simulink model "SystummThinkers_Simulink"  (R2025a)
settings: Solver=VariableStepAuto  StartTime=0.0  StopTime=50  RelTol=1e-3
libraries: slpidlib x2
settings Model: Creator=mostlyk  LastModifiedBy=Anish Toshniwal

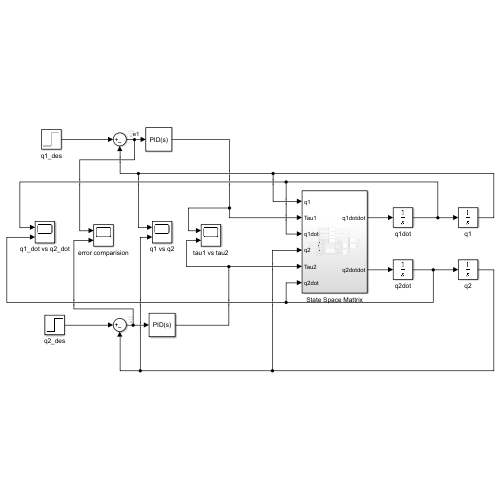
[thumbnail: Simulink's stored preview of the top-level diagram]
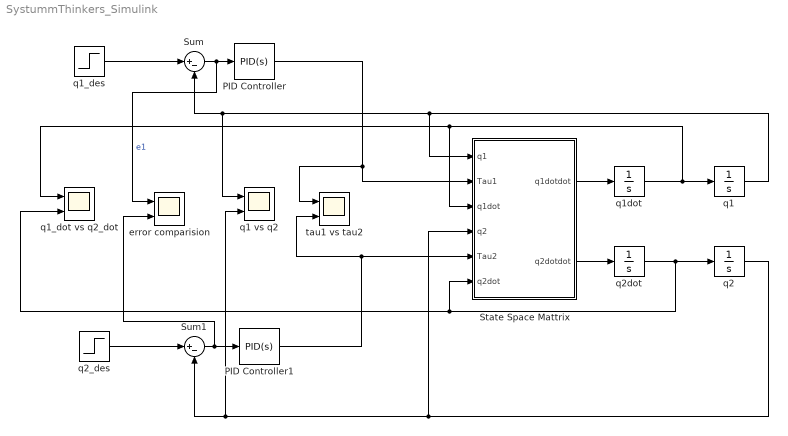
== system SystummThinkers_Simulink ==
  PID Controller : slpidlib/PID Controller  Controller=PID  Form=Parallel  TimeDomain=Continuous-time  UseExternalTs=off  SampleTime=-1  IntegratorMethod=Forward Euler  FilterMethod=Forward Euler  ControllerParametersSource=internal  P=120  I=180  UseKiTs=off  D=150  UseExternalDerivativeSource=off  N=100  UseFilter=on  TunerSelectOption=Transfer Function Based (PID Tuner App)  InitialConditionSource=internal  InitialConditionForIntegrator=0  InitialConditionForFilter=0  DifferentiatorICPrevScaledInput=0  ExternalReset=none  TrackingMode=off  Kt=1  LimitOutput=off  SatLimitsSource=internal  UpperSaturationLimit=inf  LowerSaturationLimit=-inf  LinearizeAsGain=on  AntiWindupMode=none  Kb=1  LimitIntegrator=off  UpperIntegratorSaturationLimit=inf  LowerIntegratorSaturationLimit=-inf  POutMin=[]  POutMax=[]  IOutMin=[]  IOutMax=[]  DOutMin=[]  DOutMax=[]  NOutMin=[]  NOutMax=[]  SumOutMin=[]  SumOutMax=[]  SaturationOutMin=[]  SaturationOutMax=[]  PParamMin=[]  PParamMax=[]  IParamMin=[]  IParamMax=[]  DParamMin=[]  DParamMax=[]  NParamMin=[]  NParamMax=[]  KbParamMin=[]  KbParamMax=[]  KtParamMin=[]  KtParamMax=[]  KbOutMin=[]  KbOutMax=[]  KtOutMin=[]  KtOutMax=[]  IntegratorOutMin=[]  IntegratorOutMax=[]  FilterOutMin=[]  FilterOutMax=[]  SumI1OutMin=[]  SumI1OutMax=[]  SumI2OutMin=[]  SumI2OutMax=[]  SumI3OutMin=[]  SumI3OutMax=[]  SumI4OutMin=[]  SumI4OutMax=[]  SumDOutMin=[]  SumDOutMax=[]  DifferentiatorOutMin=[]  DifferentiatorOutMax=[]  FilterDiffOutCoefMin=[]  FilterDiffOutCoefMax=[]  ReciprocalOutMin=[]  ReciprocalOutMax=[]  SumDenOutMin=[]  SumDenOutMax=[]  SumNumOutMin=[]  SumNumOutMax=[]  DivideOutMin=[]  DivideOutMax=[]  UdiffTsProdOutMin=[]  UdiffTsProdOutMax=[]  NTsProdOutMin=[]  NTsProdOutMax=[]  UintegralTsProdOutMin=[]  UintegralTsProdOutMax=[]  UngainTsProdOutMin=[]  UngainTsProdOutMax=[]  ClampingZeroOutDataTypeStr=Inherit: Inherit via back propagation  ClampingZeroOutMin=[]  ClampingZeroOutMax=[]  FilterDenConstantOutDataTypeStr=Inherit: Inherit via back propagation  FilterDenConstantOutMin=[]  FilterDenConstantOutMax=[]  PCopyOutDataTypeStr=Inherit: Inherit via back propagation  PCopyOutMin=[]  PCopyOutMax=[]  NCopyOutDataTypeStr=Inherit: Inherit via back propagation  NCopyOutMin=[]  NCopyOutMax=[]  IntegratorContinuousStateAttributes=''  IntegratorStateMustResolveToSignalObject=off  IntegratorRTWStateStorageClass=Auto  FilterContinuousStateAttributes=''  FilterStateMustResolveToSignalObject=off  FilterRTWStateStorageClass=Auto  ParallelPVariant=InternalParameters  IdealPVariant=Disabled  IVariant=InternalParameters  DVariant=InternalParameters  IntegratorVariant=Continuous  SatVariant=Disabled  AWVariant=Passthrough  PCopyVariant=Disabled  TRVariant=Disabled  FdbkBlocksVariant=Forward  IdealPFdbkVariant=Disabled  SatFdbkVariant=Disabled  DerivativeFilterVariant=ContFilter  NVariant=InternalParameters  NCopyVariant=Disabled  FilterICVariant=InternalICsFilter  IntegratorICVariant=InternalICs  ExternalResetVariant=Disabled  TRSumVariant=Passthrough  SumFdbkVariant=Disabled  SumVariant=Sum_PID  TsampFilterVariant=InternalTs  TsampNgainVariant=Passthrough  TsampIntegralVariant=Disabled_SignalSpec  ExternalSaturationOutDataTypeStr=Inherit: Same as second input  DerivativeSourceVariant=ErrorSignal  PreIntVariant=InternalPreInt
  PID Controller1 : slpidlib/PID Controller  Controller=PID  Form=Parallel  TimeDomain=Continuous-time  UseExternalTs=off  SampleTime=-1  IntegratorMethod=Forward Euler  FilterMethod=Forward Euler  ControllerParametersSource=internal  P=120  I=180  UseKiTs=off  D=150  UseExternalDerivativeSource=off  N=100  UseFilter=on  TunerSelectOption=Transfer Function Based (PID Tuner App)  InitialConditionSource=internal  InitialConditionForIntegrator=0  InitialConditionForFilter=0  DifferentiatorICPrevScaledInput=0  ExternalReset=none  TrackingMode=off  Kt=1  LimitOutput=off  SatLimitsSource=internal  UpperSaturationLimit=inf  LowerSaturationLimit=-inf  LinearizeAsGain=on  AntiWindupMode=none  Kb=1  LimitIntegrator=off  UpperIntegratorSaturationLimit=inf  LowerIntegratorSaturationLimit=-inf  POutMin=[]  POutMax=[]  IOutMin=[]  IOutMax=[]  DOutMin=[]  DOutMax=[]  NOutMin=[]  NOutMax=[]  SumOutMin=[]  SumOutMax=[]  SaturationOutMin=[]  SaturationOutMax=[]  PParamMin=[]  PParamMax=[]  IParamMin=[]  IParamMax=[]  DParamMin=[]  DParamMax=[]  NParamMin=[]  NParamMax=[]  KbParamMin=[]  KbParamMax=[]  KtParamMin=[]  KtParamMax=[]  KbOutMin=[]  KbOutMax=[]  KtOutMin=[]  KtOutMax=[]  IntegratorOutMin=[]  IntegratorOutMax=[]  FilterOutMin=[]  FilterOutMax=[]  SumI1OutMin=[]  SumI1OutMax=[]  SumI2OutMin=[]  SumI2OutMax=[]  SumI3OutMin=[]  SumI3OutMax=[]  SumI4OutMin=[]  SumI4OutMax=[]  SumDOutMin=[]  SumDOutMax=[]  DifferentiatorOutMin=[]  DifferentiatorOutMax=[]  FilterDiffOutCoefMin=[]  FilterDiffOutCoefMax=[]  ReciprocalOutMin=[]  ReciprocalOutMax=[]  SumDenOutMin=[]  SumDenOutMax=[]  SumNumOutMin=[]  SumNumOutMax=[]  DivideOutMin=[]  DivideOutMax=[]  UdiffTsProdOutMin=[]  UdiffTsProdOutMax=[]  NTsProdOutMin=[]  NTsProdOutMax=[]  UintegralTsProdOutMin=[]  UintegralTsProdOutMax=[]  UngainTsProdOutMin=[]  UngainTsProdOutMax=[]  ClampingZeroOutDataTypeStr=Inherit: Inherit via back propagation  ClampingZeroOutMin=[]  ClampingZeroOutMax=[]  FilterDenConstantOutDataTypeStr=Inherit: Inherit via back propagation  FilterDenConstantOutMin=[]  FilterDenConstantOutMax=[]  PCopyOutDataTypeStr=Inherit: Inherit via back propagation  PCopyOutMin=[]  PCopyOutMax=[]  NCopyOutDataTypeStr=Inherit: Inherit via back propagation  NCopyOutMin=[]  NCopyOutMax=[]  IntegratorContinuousStateAttributes=''  IntegratorStateMustResolveToSignalObject=off  IntegratorRTWStateStorageClass=Auto  FilterContinuousStateAttributes=''  FilterStateMustResolveToSignalObject=off  FilterRTWStateStorageClass=Auto  ParallelPVariant=InternalParameters  IdealPVariant=Disabled  IVariant=InternalParameters  DVariant=InternalParameters  IntegratorVariant=Continuous  SatVariant=Disabled  AWVariant=Passthrough  PCopyVariant=Disabled  TRVariant=Disabled  FdbkBlocksVariant=Forward  IdealPFdbkVariant=Disabled  SatFdbkVariant=Disabled  DerivativeFilterVariant=ContFilter  NVariant=InternalParameters  NCopyVariant=Disabled  FilterICVariant=InternalICsFilter  IntegratorICVariant=InternalICs  ExternalResetVariant=Disabled  TRSumVariant=Passthrough  SumFdbkVariant=Disabled  SumVariant=Sum_PID  TsampFilterVariant=InternalTs  TsampNgainVariant=Passthrough  TsampIntegralVariant=Disabled_SignalSpec  ExternalSaturationOutDataTypeStr=Inherit: Same as second input  DerivativeSourceVariant=ErrorSignal  PreIntVariant=InternalPreInt
  State Space Mattrix : Subsystem
  Sum : Sum  Inputs=|+-
  Sum1 : Sum  Inputs=|+-
  error comparision : Scope  NumInputPorts=2
      settings: ActiveDisplayYMinimum=-1  ActiveDisplayYMaximum=1
  q1 : Integrator  InitialCondition=0.1
  q1 vs q2 : Scope  NumInputPorts=2
      settings: ActiveDisplayYMinimum=-0.27365843091544217  ActiveDisplayYMaximum=0.20860466599804511
  q1_des : Step  After=0  SampleTime=0
  q1_dot vs q2_dot : Scope  NumInputPorts=2
      settings: ActiveDisplayYMinimum=-16.221672111581775  ActiveDisplayYMaximum=9.3160134029449342  DataLoggingVariableName=ScopeData2
  q1dot : Integrator
  q2 : Integrator  InitialCondition=0.1
  q2_des : Step  After=0  SampleTime=0
  q2dot : Integrator
  tau1 vs tau2 : Scope  NumInputPorts=2
      settings: ActiveDisplayYMinimum=-30.7924543124781  ActiveDisplayYMaximum=40.414840154467996  DataLoggingVariableName=ScopeData3
  wires:
  q1/1 -> State Space Mattrix/1(q1), Sum/2, q1 vs q2/1
  Sum/1 -> PID Controller/1, error comparision/1  "e1"
  q1_des/1 -> Sum/1
  q1dot/1 -> q1_dot vs q2_dot/1, State Space Mattrix/3(q1dot), q1/1
  PID Controller/1 -> tau1 vs tau2/1, State Space Mattrix/2(Tau1)
  q2_des/1 -> Sum1/1
  q2/1 -> Sum1/2, q1 vs q2/2, State Space Mattrix/4(q2)
  State Space Mattrix/2(q2dotdot) -> q2dot/1
  q2dot/1 -> q2/1, q1_dot vs q2_dot/2, State Space Mattrix/6(q2dot)
  PID Controller1/1 -> tau1 vs tau2/2, State Space Mattrix/5(Tau2)
  State Space Mattrix/1(q1dotdot) -> q1dot/1
  Sum1/1 -> error comparision/2, PID Controller1/1

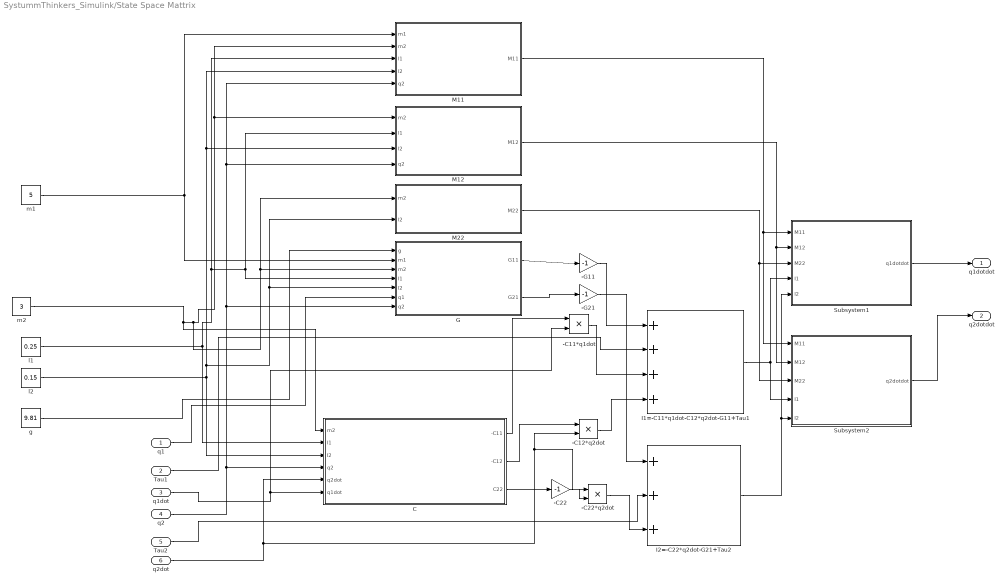
== system SystummThinkers_Simulink/State Space Mattrix ==
  q1 : Inport
  Tau1 : Inport  Port=2
  q1dot : Inport  Port=3
  q2 : Inport  Port=4
  Tau2 : Inport  Port=5
  q2dot : Inport  Port=6
  -C11*q1dot : Product
  -C12*q2dot : Product
  -C22 : Gain  Gain=-1
  -C22*q2dot : Product
  -G11 : Gain  Gain=-1
  -G21 : Gain  Gain=-1
  C : Subsystem
  G : Subsystem
  I1=-C11*q1dot-C12*q2dot-G11+Tau1 : Sum  Inputs=++++
  I2=-C22*q2dot-G21+Tau2 : Sum  Inputs=+++
  M11 : Subsystem
  M12 : Subsystem
  M22 : Subsystem
  Subsystem1 : Subsystem
  Subsystem2 : Subsystem
  g : Constant  Value=9.81
  l1 : Constant  Value=0.25
  l2 : Constant  Value=0.15
  m1 : Constant  Value=5
  m2 : Constant  Value=3
  q1dotdot : Outport
  q2dotdot : Outport  Port=2
  wires:
  m1/1 -> G/2(m1), M11/1(m1)
  m2/1 -> C/1(m2), M22/1(m2), G/3(m2), M11/2(m2), M12/1(m2)
  l1/1 -> C/2(l1), M11/3(l1), G/4(l1), M12/2(l1)
  l2/1 -> C/3(I2), M22/2(l2), G/5(l2), M11/4(l2), M12/3(l2)
  q2/1 -> M11/5(q2), M12/4(q2), G/7(q2), C/4(q2)
  q1/1 -> G/6(q1)
  g/1 -> G/1(g)
  q2dot/1 -> C/5(q2dot), -C12*q2dot/2, -C22*q2dot/1
  q1dot/1 -> -C11*q1dot/2, C/6(q1dot)
  C/1(-C11) -> -C11*q1dot/1
  C/2(-C12) -> -C12*q2dot/1
  G/1(G11) -> -G11/1
  -C12*q2dot/1 -> I1=-C11*q1dot-C12*q2dot-G11+Tau1/4
  -C11*q1dot/1 -> I1=-C11*q1dot-C12*q2dot-G11+Tau1/3
  -G11/1 -> I1=-C11*q1dot-C12*q2dot-G11+Tau1/1
  Tau1/1 -> I1=-C11*q1dot-C12*q2dot-G11+Tau1/2
  C/3(C22) -> -C22/1
  -C22/1 -> -C22*q2dot/2
  G/2(G21) -> -G21/1
  -C22*q2dot/1 -> I2=-C22*q2dot-G21+Tau2/3
  -G21/1 -> I2=-C22*q2dot-G21+Tau2/1
  Tau2/1 -> I2=-C22*q2dot-G21+Tau2/2
  M11/1(M11) -> Subsystem2/1(M11), Subsystem1/1(M11)
  M12/1(M12) -> Subsystem2/2(M12), Subsystem1/2(M12)
  M22/1(M22) -> Subsystem2/3(M22), Subsystem1/3(M22)
  I1=-C11*q1dot-C12*q2dot-G11+Tau1/1 -> Subsystem1/4(I1), Subsystem2/4(I1)
  I2=-C22*q2dot-G21+Tau2/1 -> Subsystem1/5(I2), Subsystem2/5(I2)
  Subsystem1/1("q1dotdot ") -> q1dotdot/1
  Subsystem2/1("q2dotdot ") -> q2dotdot/1

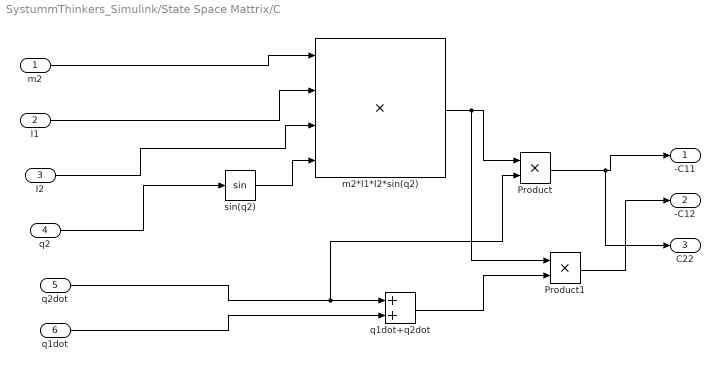
== system SystummThinkers_Simulink/State Space Mattrix/C ==
  m2 : Inport
  l1 : Inport  Port=2
  I2 : Inport  Port=3
  q2 : Inport  Port=4
  q2dot : Inport  Port=5
  q1dot : Inport  Port=6
  Product : Product
  Product1 : Product
  m2*l1*l2*sin(q2) : Product  Inputs=4
  q1dot+q2dot : Sum
  sin(q2) : Trigonometry
  -C11 : Outport
  -C12 : Outport  Port=2
  C22 : Outport  Port=3
  wires:
  q2/1 -> sin(q2)/1
  sin(q2)/1 -> m2*l1*l2*sin(q2)/4
  m2/1 -> m2*l1*l2*sin(q2)/1
  l1/1 -> m2*l1*l2*sin(q2)/2
  I2/1 -> m2*l1*l2*sin(q2)/3
  q1dot/1 -> q1dot+q2dot/2
  q2dot/1 -> Product/2, q1dot+q2dot/1
  m2*l1*l2*sin(q2)/1 -> Product1/1, Product/1
  Product/1 -> C22/1, -C11/1
  q1dot+q2dot/1 -> Product1/2
  Product1/1 -> -C12/1

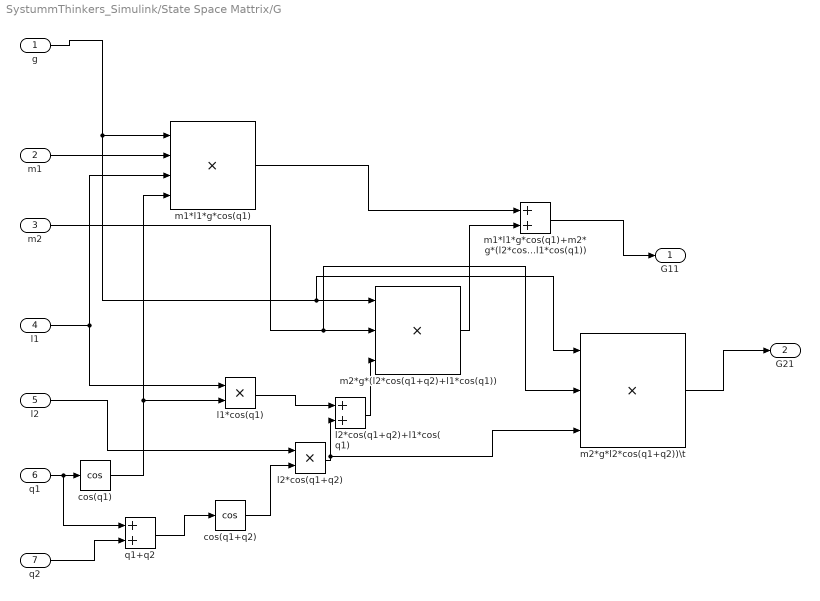
== system SystummThinkers_Simulink/State Space Mattrix/G ==
  g : Inport
  m1 : Inport  Port=2
  m2 : Inport  Port=3
  l1 : Inport  Port=4
  l2 : Inport  Port=5
  q1 : Inport  Port=6
  q2 : Inport  Port=7
  cos(q1) : Trigonometry  Operator=cos
  cos(q1+q2) : Trigonometry  Operator=cos
  l1*cos(q1) : Product
  l2*cos(q1+q2) : Product
  l2*cos(q1+q2)+l1*cos(q1) : Sum
  m1*l1*g*cos(q1) : Product  Inputs=4
  m1*l1*g*cos(q1)+m2*g*(l2*cos(q1+q2)+l1*cos(q1)) : Sum
  m2*g*(l2*cos(q1+q2)+l1*cos(q1)) : Product  Inputs=3
  m2*g*l2*cos(q1+q2))\t : Product  Inputs=3
  q1+q2 : Sum
  G11 : Outport
  G21 : Outport  Port=2
  wires:
  q1/1 -> q1+q2/1, cos(q1)/1
  g/1 -> m2*g*l2*cos(q1+q2))\t/1, m2*g*(l2*cos(q1+q2)+l1*cos(q1))/1, m1*l1*g*cos(q1)/1
  m1/1 -> m1*l1*g*cos(q1)/2
  l1/1 -> l1*cos(q1)/1, m1*l1*g*cos(q1)/3
  cos(q1)/1 -> l1*cos(q1)/2, m1*l1*g*cos(q1)/4
  q2/1 -> q1+q2/2
  q1+q2/1 -> cos(q1+q2)/1
  cos(q1+q2)/1 -> l2*cos(q1+q2)/2
  l2/1 -> l2*cos(q1+q2)/1
  l2*cos(q1+q2)/1 -> m2*g*l2*cos(q1+q2))\t/3, l2*cos(q1+q2)+l1*cos(q1)/2
  l1*cos(q1)/1 -> l2*cos(q1+q2)+l1*cos(q1)/1
  l2*cos(q1+q2)+l1*cos(q1)/1 -> m2*g*(l2*cos(q1+q2)+l1*cos(q1))/3
  m2/1 -> m2*g*(l2*cos(q1+q2)+l1*cos(q1))/2, m2*g*l2*cos(q1+q2))\t/2
  m1*l1*g*cos(q1)/1 -> m1*l1*g*cos(q1)+m2*g*(l2*cos(q1+q2)+l1*cos(q1))/1
  m2*g*(l2*cos(q1+q2)+l1*cos(q1))/1 -> m1*l1*g*cos(q1)+m2*g*(l2*cos(q1+q2)+l1*cos(q1))/2
  m1*l1*g*cos(q1)+m2*g*(l2*cos(q1+q2)+l1*cos(q1))/1 -> G11/1
  m2*g*l2*cos(q1+q2))\t/1 -> G21/1

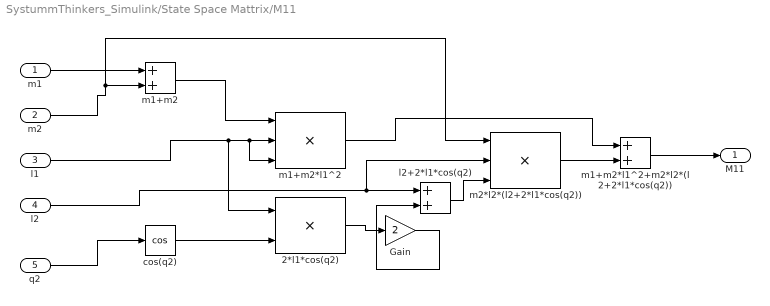
== system SystummThinkers_Simulink/State Space Mattrix/M11 ==
  m1 : Inport
  m2 : Inport  Port=2
  l1 : Inport  Port=3
  l2 : Inport  Port=4
  q2 : Inport  Port=5
  2*l1*cos(q2) : Product
  Gain : Gain  Gain=2
  cos(q2) : Trigonometry  Operator=cos
  l2+2*l1*cos(q2) : Sum
  m1+m2 : Sum
  m1+m2*l1^2 : Product  Inputs=3
  m1+m2*l1^2+m2*l2*(l2+2*l1*cos(q2)) : Sum
  m2*l2*(l2+2*l1*cos(q2)) : Product  Inputs=3
  M11 : Outport
  wires:
  m1/1 -> m1+m2/1
  m2/1 -> m2*l2*(l2+2*l1*cos(q2))/1, m1+m2/2
  m1+m2/1 -> m1+m2*l1^2/1
  l1/1 -> 2*l1*cos(q2)/1, m1+m2*l1^2/3, m1+m2*l1^2/2
  q2/1 -> cos(q2)/1
  cos(q2)/1 -> 2*l1*cos(q2)/2
  l2/1 -> m2*l2*(l2+2*l1*cos(q2))/2, l2+2*l1*cos(q2)/1
  l2+2*l1*cos(q2)/1 -> m2*l2*(l2+2*l1*cos(q2))/3
  m2*l2*(l2+2*l1*cos(q2))/1 -> m1+m2*l1^2+m2*l2*(l2+2*l1*cos(q2))/2
  m1+m2*l1^2/1 -> m1+m2*l1^2+m2*l2*(l2+2*l1*cos(q2))/1
  m1+m2*l1^2+m2*l2*(l2+2*l1*cos(q2))/1 -> M11/1
  2*l1*cos(q2)/1 -> Gain/1
  Gain/1 -> l2+2*l1*cos(q2)/2

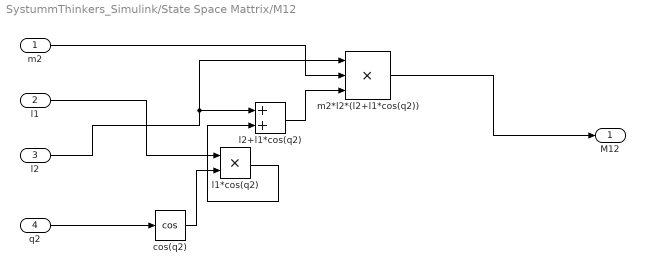
== system SystummThinkers_Simulink/State Space Mattrix/M12 ==
  m2 : Inport
  l1 : Inport  Port=2
  l2 : Inport  Port=3
  q2 : Inport  Port=4
  cos(q2) : Trigonometry  Operator=cos
  l1*cos(q2) : Product
  l2+l1*cos(q2) : Sum
  m2*l2*(l2+l1*cos(q2)) : Product  Inputs=3
  M12 : Outport
  wires:
  q2/1 -> cos(q2)/1
  l1/1 -> l1*cos(q2)/1
  cos(q2)/1 -> l1*cos(q2)/2
  l1*cos(q2)/1 -> l2+l1*cos(q2)/2
  l2/1 -> m2*l2*(l2+l1*cos(q2))/1, l2+l1*cos(q2)/1
  l2+l1*cos(q2)/1 -> m2*l2*(l2+l1*cos(q2))/3
  m2/1 -> m2*l2*(l2+l1*cos(q2))/2
  m2*l2*(l2+l1*cos(q2))/1 -> M12/1

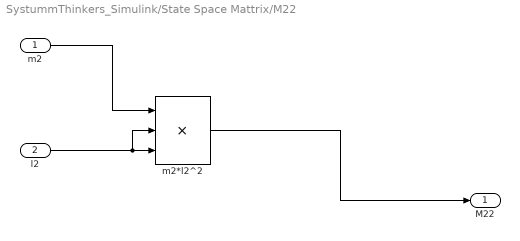
== system SystummThinkers_Simulink/State Space Mattrix/M22 ==
  m2 : Inport
  l2 : Inport  Port=2
  m2*l2^2 : Product  Inputs=3
  M22 : Outport
  wires:
  m2/1 -> m2*l2^2/1
  l2/1 -> m2*l2^2/2, m2*l2^2/3
  m2*l2^2/1 -> M22/1

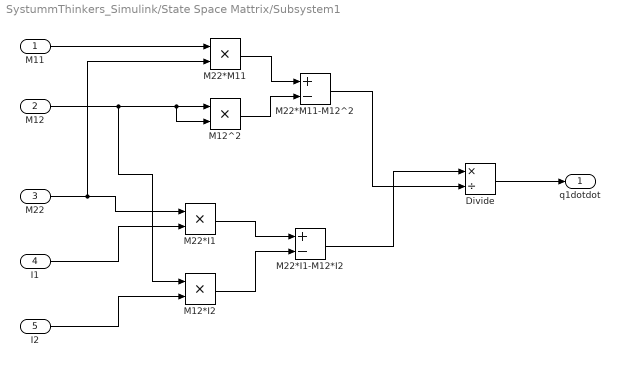
== system SystummThinkers_Simulink/State Space Mattrix/Subsystem1 ==
  M11 : Inport
  M12 : Inport  Port=2
  M22 : Inport  Port=3
  I1 : Inport  Port=4
  I2 : Inport  Port=5
  Divide : Product  Inputs=*/
  M12*I2 : Product
  M12^2 : Product
  M22*I1 : Product
  M22*I1-M12*I2 : Sum  Inputs=+-
  M22*M11 : Product
  M22*M11-M12^2 : Sum  Inputs=+-
  "q1dotdot " : Outport
  wires:
  M22/1 -> M22*M11/2, M22*I1/1
  I1/1 -> M22*I1/2
  M12/1 -> M12^2/2, M12^2/1, M12*I2/1
  I2/1 -> M12*I2/2
  M22*I1/1 -> M22*I1-M12*I2/1
  M12*I2/1 -> M22*I1-M12*I2/2
  M11/1 -> M22*M11/1
  M22*M11/1 -> M22*M11-M12^2/1
  M12^2/1 -> M22*M11-M12^2/2
  M22*I1-M12*I2/1 -> Divide/1
  M22*M11-M12^2/1 -> Divide/2
  Divide/1 -> "q1dotdot "/1

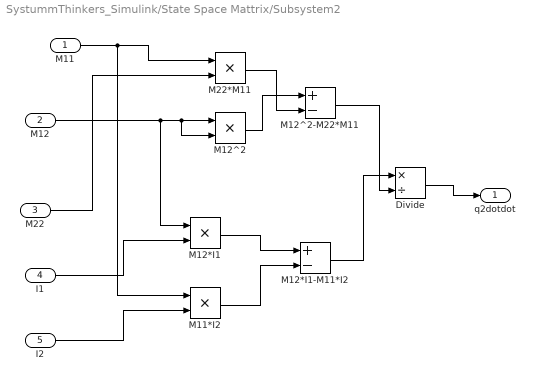
== system SystummThinkers_Simulink/State Space Mattrix/Subsystem2 ==
  M11 : Inport
  M12 : Inport  Port=2
  M22 : Inport  Port=3
  I1 : Inport  Port=4
  I2 : Inport  Port=5
  Divide : Product  Inputs=*/
  M11*I2 : Product
  M12*I1 : Product
  M12*I1-M11*I2 : Sum  Inputs=+-
  M12^2 : Product
  M12^2-M22*M11 : Sum  Inputs=+-
  M22*M11 : Product
  "q2dotdot " : Outport
  wires:
  M22/1 -> M22*M11/2
  I1/1 -> M12*I1/2
  M12/1 -> M12*I1/1, M12^2/2, M12^2/1
  I2/1 -> M11*I2/2
  M12*I1/1 -> M12*I1-M11*I2/1
  M11*I2/1 -> M12*I1-M11*I2/2
  M11/1 -> M11*I2/1, M22*M11/1
  M12*I1-M11*I2/1 -> Divide/1
  M12^2-M22*M11/1 -> Divide/2
  Divide/1 -> "q2dotdot "/1
  M22*M11/1 -> M12^2-M22*M11/2
  M12^2/1 -> M12^2-M22*M11/1
